simulink model "controller_model"  (R2016b)
settings: Solver=ode4  StartTime=0.0  StopTime=tend  FixedStep=dt_rths  RelTol=1e-3
values from neighbouring files (symbols this model uses):
  last_state = [0.000382206380198 -7.38093275994e-07 -1.38273003581e-05 1.96390758506e-05 4.26666429273e-06 0.174746860236 1.12144478912e-05 -1.41008002241e-05 4.85589159386e-05 5.00618389181e-06 0.00266509092567 0.0289443653817 ... (64 elements, 64x1)]    [last.mat]    (also in model.m = (1 - learning_rate) * last_state +                          )
  Po = [9760904.15347 -48101.0819174 -41991.4751638 58292.1547817 -72237.8147125 -25474.7799626 84633.4351337 -102168.900459 31909.6252909 -53126.3170596 38563.2006474 22025.636778 ... (4096 elements, 64x64)]    [Po.mat]    (also in model.m = inv(auto_corr_mue + 1e-3*eye(n_nodes, n_nodes)))
  sat_limit_lower = -3.8    [F1_input_file.m]
  sat_limit_upper = +3.8    (= 3.8)    [F1_input_file.m]
  W = [-0.130683217431 0.0603641643112 -0.00407628912708 -0.00291680233653 -0.0114941494034 0.00419260374661 0.00359952525664 0.0135569595763 -0.0120134311899 0.00841261688404 -0.0783948215385 -0.00315849787389 ... (4096 elements, 64x64)]    [W.mat]    (also in model.m = zeros(n_nodes))
  W_in = zeros(n_nodes, n_input)    [model.m]    (also in w_in.mat = [0 0 0 0 0 0 0 0 0 0 0 0 ... (64 elements, 64x1)])
  W_out = [1.20598770721 0.151528546652 0.275191372784 0.064836724152 -1.2476406116 -0.116141380102 0.55238421628 4.40846307715 -2.93771661486 -0.875752742868 -0.0118066638097 0.696309987921 ... (64 elements, 1x64)]    [W_out.mat]    (also in model.m = zeros(n_output, n_nodes + n_input - 1))
libraries: simulink x1
settings Model: Creator=Sandra  LastModifiedBy=wal26
settings DataIOCC: SaveFormat=StructureWithTime
settings OptimizationCC: LifeSpan=inf
settings DebuggingCC: InheritedTsInSrcMsg=none  SFExecutionAtInitializationDiag=none
settings HardwareCC: ProdBitPerSizeT=32  ProdBitPerPtrDiffT=32  ProdWordSize=32  ProdHWDeviceType=Specified
settings ModelReferenceCC: ModelReferenceNumInstancesAllowed=Single

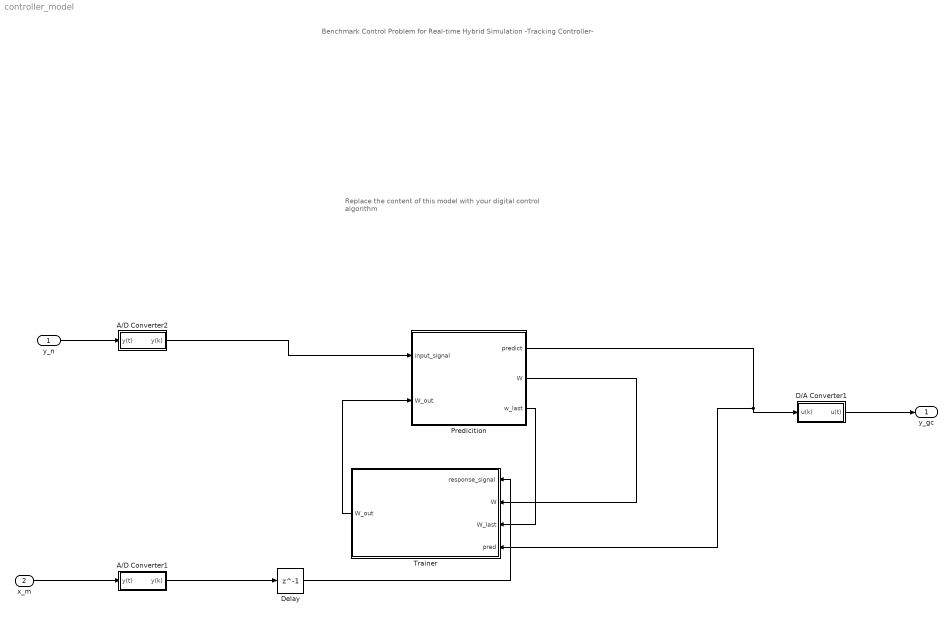
== system controller_model ==
  note: Benchmark Control Problem for Real-time Hybrid Simulation
      | -Tracking Controller-
  note: Replace the content of this model
      | with your digital control algorithm
  y_n : Inport
  x_m : Inport  Port=2
  A/D Converter1 : Subsystem
  A/D Converter2 : Subsystem
  D/A Converter1 : Subsystem
  Delay : Delay  DelayLength=1
  Predicition : Subsystem
  Trainer : Subsystem
  y_gc : Outport
  wires:
  Trainer/1(W_out) -> Predicition/2(W_out)
  Predicition/2(W) -> Trainer/2(W)
  x_m/1 -> A/D Converter1/1(y(t))
  D/A Converter1/1(u(t)) -> y_gc/1
  Predicition/3(w_last) -> Trainer/3(W_last)
  Predicition/1(predict) -> Trainer/4(pred), D/A Converter1/1(u(k))
  y_n/1 -> A/D Converter2/1(y(t))
  A/D Converter1/1(y(k)) -> Delay/1
  A/D Converter2/1(y(k)) -> Predicition/1(input_signal)
  Delay/1 -> Trainer/1(response_signal)

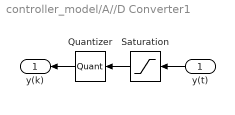
== system controller_model/A//D Converter1 ==
  y(t) : Inport
  Quantizer : Quantizer  QuantizationInterval=quantize_int
  Saturation : Saturate  UpperLimit=sat_limit_upper  LowerLimit=sat_limit_lower
  y(k) : Outport
  wires:
  Saturation/1 -> Quantizer/1
  Quantizer/1 -> y(k)/1
  y(t)/1 -> Saturation/1

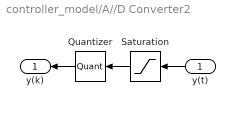
== system controller_model/A//D Converter2 ==
  y(t) : Inport
  Quantizer : Quantizer  QuantizationInterval=quantize_int
  Saturation : Saturate  UpperLimit=sat_limit_upper  LowerLimit=sat_limit_lower
  y(k) : Outport
  wires:
  Saturation/1 -> Quantizer/1
  Quantizer/1 -> y(k)/1
  y(t)/1 -> Saturation/1

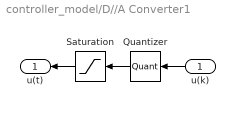
== system controller_model/D//A Converter1 ==
  u(k) : Inport
  Quantizer : Quantizer  QuantizationInterval=quantize_int
  Saturation : Saturate  UpperLimit=sat_limit_upper  LowerLimit=sat_limit_lower
  u(t) : Outport
  wires:
  Saturation/1 -> u(t)/1
  Quantizer/1 -> Saturation/1
  u(k)/1 -> Quantizer/1

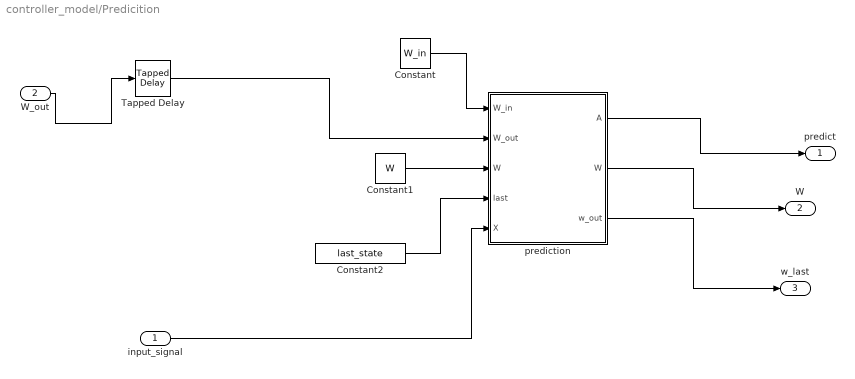
== system controller_model/Predicition ==
  input_signal : Inport
  W_out : Inport  Port=2
  Constant : Constant  Value=W_in
  Constant1 : Constant  Value=W
  Constant2 : Constant  Value=last_state
  Tapped Delay : simulink/Discrete/Tapped Delay  vinit=W_out  samptime=-1  NumDelays=1  DelayOrder=Oldest  includeCurrent=off
  prediction : MATLAB Function  TreatAsAtomicUnit=on
  predict : Outport
  W : Outport  Port=2
  w_last : Outport  Port=3
  wires:
  W_out/1 -> Tapped Delay/1
  prediction/1(A) -> predict/1
  input_signal/1 -> prediction/5(X)
  Constant/1 -> prediction/1(W_in)
  Constant1/1 -> prediction/3("W ")
  Constant2/1 -> prediction/4(last)
  Tapped Delay/1 -> prediction/2(W_out)
  prediction/2(W) -> W/1
  prediction/3(w_out) -> w_last/1

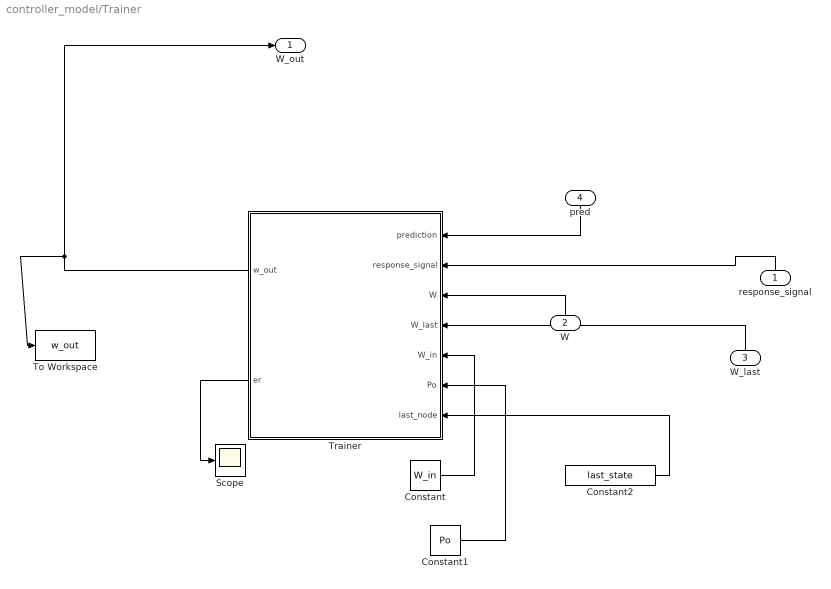
== system controller_model/Trainer ==
  response_signal : Inport
  W : Inport  Port=2
  W_last : Inport  Port=3
  pred : Inport  Port=4
  Constant : Constant  Value=W_in
  Constant1 : Constant  Value=Po
  Constant2 : Constant  Value=last_state
  Scope : Scope
  To Workspace : ToWorkspace  VariableName=w_out  SaveFormat=Timeseries  SampleTime=-1
  Trainer : MATLAB Function  TreatAsAtomicUnit=on
  W_out : Outport
  wires:
  Trainer/1(w_out) -> To Workspace/1, W_out/1
  Trainer/2(er) -> Scope/1
  W/1 -> Trainer/3(W)
  W_last/1 -> Trainer/4(W_last)
  pred/1 -> Trainer/1(prediction)
  Constant/1 -> Trainer/5(W_in)
  Constant1/1 -> Trainer/6(Po)
  response_signal/1 -> Trainer/2(response_signal)
  Constant2/1 -> Trainer/7(last_node)

== matlab function controller_model/Predicition/prediction ==
  data: W_in input; W_out input; W input; last input; X input; A output; W output; w_out output
function [A, W, w_out]  = fcn(W_in, W_out, W, last, X)

    persistent last_state;
    if isempty(last_state)
        last_state = last;
    end
    lr = 0.95;

    W_in = reshape(W_in,64,1);
    W_out = reshape(W_out, 1, 64);
    W = reshape(W, 64, 64);
     last = reshape(last,64,1);
     w_out = W_out;
    persistent node_last
    persistent init
    if isempty(node_last) && isempty(init)
        node_last = zeros(size(last));
        node_last(:) = last;
        init = 0;
    end
    U = X;
    node_updates = tanh(W_in * U + W * node_last);
    node_last = (1-lr)*node_last + lr .* node_updates;
    
    if(init == 0)
        y_predict = X;
    else
        y_predict = W_out * node_last;
    end
    
    A = y_predict(1);
    W = W;

    init = 1;
end

== matlab function controller_model/Trainer/Trainer ==
  data: prediction input; response_signal input; W input; w_out output; W_last input; er output; W_in input; Po input; last_node input
function [w_out, er]   = fcn(prediction, response_signal,W, W_last, W_in,Po,last_node)
    persistent Pk;
    persistent node_last_adp;
    persistent time;
    persistent init;
    if(isempty(Pk) && isempty(node_last_adp) && isempty(time) && isempty(init))
        Pk = Po;
        node_last_adp = zeros(64,1);
        node_last_adp(:) = last_node;
        time = 0;
        init = 0;
    end
    lr = 0.95;
    
    %send response to reservoir for to do the comparation
    node = tanh(W_in * response_signal + W * node_last_adp);
    node_last_adp = (1-lr)*node_last_adp + lr .* node;

    y_predict = W_last * node_last_adp;

    
    e = prediction - y_predict;
    lambda = 0.999945; 
    
    
   
     last_node = node_last_adp';
     der = last_node*Pk;
     iz = Pk * last_node';
     cuadratic = last_node*iz;
     Pk = (1/lambda)*(Pk - iz*inv(lambda + cuadratic)*der); 
     w_out = W_last + 1*(Pk*last_node'*e)';
    
        
    er = e;
    
    time = time + 1;
    
end
